simulink model "MPU6050_acq_sf_n"  (R2024b)
settings: Solver=FixedStepAuto  StartTime=0.0  StopTime=inf  RelTol=1e-3
libraries: arduinolib x2
settings Model: ExtModeTrigDuration=2  Creator=Marc  LastModifiedBy=Nitesh
settings SolverCC: AutoInsertRateTranBlk=on
settings OptimizationCC: BlockReduction=off  BooleanDataType=off  EnhancedBackFolding=on  PassReuseOutputArgsAs=Individual arguments  ZeroExternalMemoryAtStartup=off  ZeroInternalMemoryAtStartup=off  MaxStackSize=64  OptimizeBlockOrder=speed  DifferentSizesBufferReuse=on  OptimizationCustomize=off  EfficientTunableParamExpr=on
settings DebuggingCC: SaveWithParameterizedLinksMsg=none  UnderspecifiedInitializationDetection=Classic  MergeDetectMultiDrivingBlocksExec=none  SignalResolutionControl=TryResolveAllWithWarning  ParameterTunabilityLossMsg=error
settings HardwareCC: ProdBitPerPointer=32  ProdBitPerSizeT=32  ProdBitPerPtrDiffT=32  ProdLargestAtomicInteger=Long  ProdLargestAtomicFloat=Double  ProdWordSize=32  ProdHWDeviceType=ARM Compatible->ARM Cortex  TargetIntDivRoundTo=Zero  TargetEndianess=LittleEndian  TargetHWDeviceType=Custom Processor->Custom Processor  ProdEqTarget=off  UseEmbeddedCoderFeatures=off
settings ModelReferenceCC: PropagateSignalLabelsOutOfModel=off
settings SFSimCC: MATLABDynamicMemAlloc=off
settings RTWCC: Description=Embedded Coder  SystemTargetFile=ert.tlc  HardwareBoard=ESP32-WROOM(Arduino Compatible)  TLCOptions="-aInlineSetEventsForThisBaseRateFcn=TLC_FALSE -aSuppressMultiTaskScheduler=TLC_FALSE  -aRateBasedStepFcn=0"  TemplateMakefile=ert_default_tmf  Toolchain=ESP32
settings CodeAppCC: ForceParamTrailComments=on  IgnoreCustomStorageClasses=off  OperatorAnnotations=on  SimulinkDataObjDesc=on  SFDataObjDesc=on  InsertBlockDesc=on
settings ERTTargetCC: SupportContinuousTime=on  SupportNonInlinedSFcns=on  SupportVariableSizeSignals=on  ExtModeTransport=3  ExtModeStaticAlloc=on  ExtModeAutomaticAllocSize=off  ExtModeStaticAllocSize=65536  ExtModeMexFile=ext_xcp  ExtModeIntrfLevel=Level2 - Open  InlinedParameterPlacement=Hierarchical

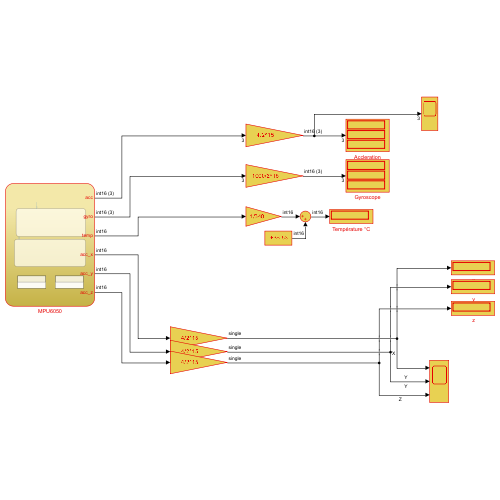
[thumbnail: Simulink's stored preview of the top-level diagram]
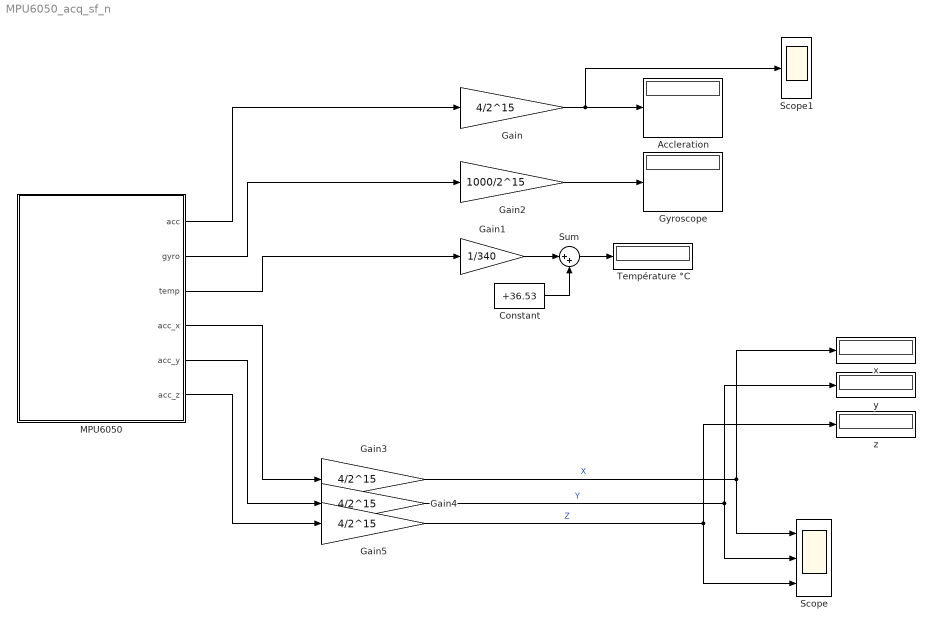
== system MPU6050_acq_sf_n ==
  " x" : Display
  " y" : Display
  " z" : Display
  Accleration : Display
  Constant : Constant  Value=+36.53  OutDataTypeStr=Inherit: Inherit via back propagation
  Gain : Gain  Gain=4/2^15  OutDataTypeStr=Inherit: Inherit via back propagation
  Gain1 : Gain  Gain=1/340  OutDataTypeStr=Inherit: Inherit via back propagation
  Gain2 : Gain  Gain=1000/2^15  OutDataTypeStr=Inherit: Inherit via back propagation
  Gain3 : Gain  Gain=4/2^15  OutDataTypeStr=single
  Gain4 : Gain  Gain=4/2^15  OutDataTypeStr=single
  Gain5 : Gain  Gain=4/2^15  OutDataTypeStr=single
  Gyroscope : Display
  MPU6050 : Stateflow chart  TreatAsAtomicUnit=on
      settings: PortSchema="{\"entries\":[{\"content\":{\"sides\":[{\"content\":{},\"type\":\"ConnectorPlacement.EquallySpacedRectSide\",\"uuid\":\"e0cad0cf-2ed8-4cf7-bff6-6ed2feffa650\"},{\"content\":{\"connectorIds\":[\"Out1\",\"Out2\",\"Out3\",\"Out4\",\"Out6\",\"Out5\"],\"side\":\"RIGHT\"},\"type\":\"ConnectorPlacement.EquallySpacedRectSide\",\"uuid\":\"9c27c799-2435-4d39-8ba1-4c3814f68cde\"},{\"content\":{\"side\":\"TOP\"},\"type\":\"ConnectorPlacement.EquallySpacedRectSide\",\"uuid\":\"52d11aab-2c42-4a19-9ee0-cf61f3e3e234\"}]},\"type\":\"ConnectorPlacement.EquallySpacedConnector\",\"uuid\":\"b37ebc91-bb9d-4b35-9b01-6a26108d89d3\"}],\"packageUris\":[\"http://schema.mathworks.com/mf0/Connector/R2020b\"],\"version\":\"1.0\"}"
  Scope : Scope  NumInputPorts=3
  Scope1 : Scope
  Sum : Sum  Inputs=|++
  Température °C : Display
  wires:
  Sum/1 -> Température °C/1
  Constant/1 -> Sum/2
  Gain1/1 -> Sum/1
  Gain2/1 -> Gyroscope/1
  MPU6050/3(temp) -> Gain1/1
  MPU6050/2(gyro) -> Gain2/1
  Gain/1 -> Scope1/1, Accleration/1
  MPU6050/1(acc) -> Gain/1
  Gain3/1 -> Scope/1, " x"/1  "X"
  Gain4/1 -> Scope/2, " y"/1  "Y"
  Gain5/1 -> " z"/1, Scope/3  "Z"
  MPU6050/4(acc_x) -> Gain3/1
  MPU6050/6(acc_y) -> Gain4/1
  MPU6050/5(acc_z) -> Gain5/1

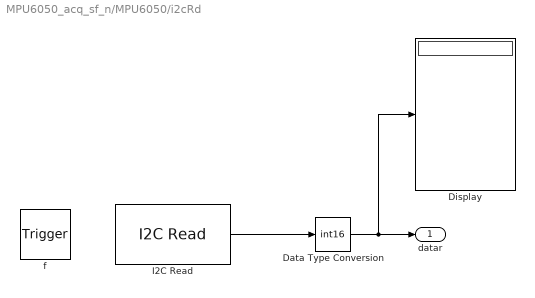
== system MPU6050_acq_sf_n/MPU6050/i2cRd ==
  f : TriggerPort  TriggerType=function-call  VariantControl=Variant  SampleTime=inf
      settings: CopyFcn=Stateflow.SLINSF.SimulinkMan.removeBlockPreDeleteFcn  PreDeleteFcn=Stateflow.SLINSF.SimulinkMan.unsafePredeleteFcn
  Data Type Conversion : DataTypeConversion  OutDataTypeStr=int16  SaturateOnIntegerOverflow=off  RndMeth=Floor
  Display : Display
  I2C Read : arduinolib/I2C Read  I2CModule=0  Mode=Master  SlaveAddress=hex2dec( '68' )  SlaveByteOrder=BigEndian  Direction=Receiver  RegisterAddressMode=on  RegisterAddress=hex2dec( '3b' )  SlaveDataType=uint16  DataLength=7  NoAck=off  RepeatedStart=off  OutputStatus=off  blockPlatform=arduino  SampleTime=-1
      settings: SourceProductName=Common
  datar : Outport  OutDataTypeStr=int16  Unit=1  PortDimensions=7  VectorParamsAs1DForOutWhenUnconnected=off
  wires:
  I2C Read/1 -> Data Type Conversion/1
  Data Type Conversion/1 -> Display/1, datar/1

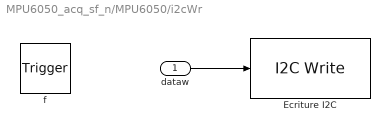
== system MPU6050_acq_sf_n/MPU6050/i2cWr ==
  dataw : Inport  OutDataTypeStr=uint16  Unit=1  PortDimensions=1
  f : TriggerPort  TriggerType=function-call  VariantControl=Variant  SampleTime=-1
      settings: CopyFcn=Stateflow.SLINSF.SimulinkMan.removeBlockPreDeleteFcn  PreDeleteFcn=Stateflow.SLINSF.SimulinkMan.unsafePredeleteFcn
  Ecriture I2C : arduinolib/I2C Write  Priority=1  I2CModule=0  Mode=Master  SlaveAddress=hex2dec( '68' )  SlaveByteOrder=BigEndian  Direction=Transmitter  RegisterAddressMode=off  RegisterAddress=hex2dec( '6B' )  SlaveDataType=uint16  DataLength=1  NoAck=off  RepeatedStart=off  OutputStatus=off  blockPlatform=arduino
      settings: SourceProductName=Common
  wires:
  dataw/1 -> Ecriture I2C/1

== stateflow chart MPU6050_acq_sf_n/MPU6050 ==
  state initialisation
    en:
    i2cWr(uint16(hex2dec( '6B00' )));%Power on
    i2cWr(uint16(hex2dec( '1B10' )));%gyro 0x10=1000°/s
    i2cWr(uint16(hex2dec( '1C08' )));%acce 0x08= 4G
    i2cWr(uint16(hex2dec( '1A06' )));%filtrage+actu 0x06= 19ms
    i2cWr(uint16(hex2dec( '3710' )));%INT_PIN_CFG
    i2cWr(uint16(hex2dec( '3800' )));%Interrupt Enable 0 désactivé
  state Lecture_acceleration3_axes
    during:
    val=i2cRd;
    acc=val(1:3);
    acc_x=val(1:1);
    acc_y=val(2:2);
    acc_z=val(3:3);
    gyro=val(5:7);
    temp=val(4:4);
  state i2cWr(dataw) [function]
  state datar = i2cRd [function]
  (default) -> initialisation
  initialisation -> Lecture_acceleration3_axes
  data: dataw function_input uint16 size=1; datar function_output int16 size=7; acc output int16 size=3; gyro output int16 size=3; val local int16 size=7; temp output int16 size=1; acc_x output; acc_z output; acc_y output
